simulink model "Second_AGC"  (R2022a)
settings: Solver=FixedStepDiscrete  StartTime=0.0  StopTime=Time*20000  RelTol=1e-3
PreLoadFcn:
  | clc,clear,close all
  | 
  | F               = 1e1;
  | Fs              = 200e6;
  | Frame           = 1  ;
  | Amplitudes      = [0.1,1,0.5,1,0.25];
  | R               = 2;
  | a               = 0.01;
  | alpha           = 0.4;
  | NumFrames       = length(Amplitudes);
  | SamplesY        = [];
  | TimeAxis        = [];
  | NumSym          = 1e3;
  | NumBitsInSymbol = 4;
  | sps             = 4;
  | rolloff         = 0.3;
  | span            = 32;
  | 
  | SQRRC = rcosdesign(rolloff, span, sps);
  | delay = mean(grpdelay(SQRRC));
  | for i = 1:NumFrames
  |     x = randi([0 3],NumSym,1);
  |     QPSK   = qammod(x,NumBitsInSymbol);
  |     Signal = Amplitudes(i) * upfirdn(QPSK, SQRRC, sps);
  |      Signal(1:delay-1)     = [];
  |      Signal(end-delay+3:end) = [];
  |     SamplesY = [SamplesY; Signal];
  | end
  | SamplesY = SamplesY.';
  | FixedRe = fi(real(SamplesY),1,16,14);
  | FixedIm = fi(imag(SamplesY),1,16,14);
  | FixedR  = fi(R,0,2,0);
  | Fixeda  = fi(a,1,13,12);
  | RealSimpleAGC = real(SamplesY);
  | ImagSimpleAGC = imag(SamplesY);
InitFcn:
  | Time = 40;
  | PowerDelay = Time*100;
libraries: sim_stud_lib_r2022a x25, dspsrcs4 x14, dspsigops x10, dspswit3 x5
(part 1 of 2)
settings Model: Creator=RolePups  LastModifiedBy=RolePups

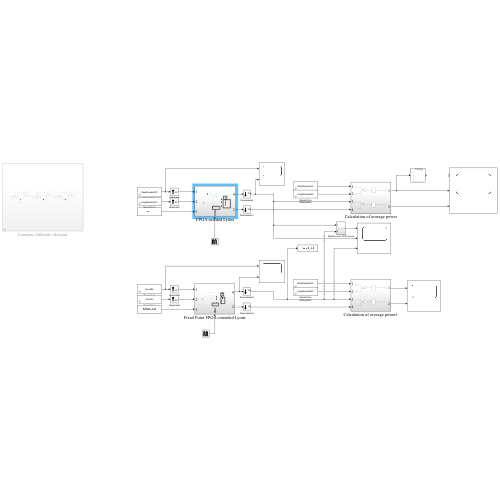
[thumbnail: Simulink's stored preview of the top-level diagram]
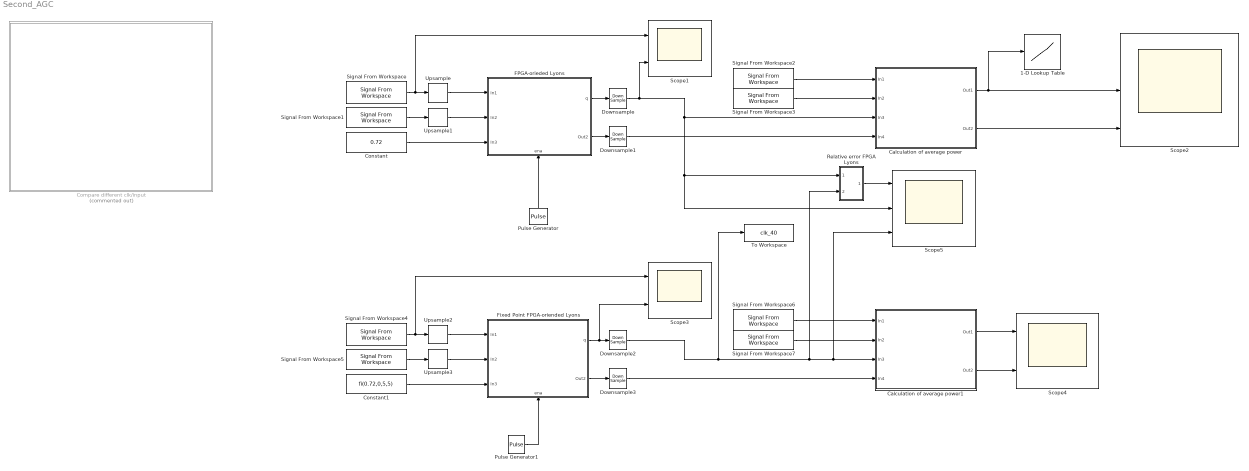
== system Second_AGC ==
  1-D Lookup Table : Lookup_n-D  NumberOfTableDimensions=1  BreakpointsForDimension1=[-5:5]  Table=10*log10([-5:5])  InternalRulePriority=Speed  RndMeth=Simplest
  Calculation of average power : Subsystem
  Calculation of average power1 : Subsystem
  Compare different clk/input : Subsystem  Commented=on
  Constant : Constant  Value=0.72
  Constant1 : Constant  Value=fi(0.72,0,5,5)
  Downsample{,1..3} (4 alike) : DownSample  N=Time  RateOptions=Allow multirate processing
  FPGA-orieded Lyons : Subsystem
      settings: PortSchema="{\"entries\":[{\"content\":{\"sides\":[{\"content\":{\"connectorIds\":[\"In1\",\"In2\",\"In3\"]},\"type\":\"ConnectorPlacement.EquallySpacedRectSide\",\"uuid\":\"2382ef4f-8b23-4fd9-9999-ae4ff3838c30\"},{\"content\":{\"connectorIds\":[\"Out1\",\"Out2\"],\"side\":\"RIGHT\"},\"type\":\"ConnectorPlacement.EquallySpacedRectSide\",\"uuid\":\"ff744322-ad90-46d9-948c-0637f52c7b9c\"},{\"content\":{\"connectorIds\":[],\"side\":\"TOP\"},\"type\":\"ConnectorPlacement.EquallySpacedRectSide\",\"uuid\":\"b0276f26-9e78-4e39-abf6-7a1348b88309\"},{\"content\":{\"connectorIds\":[\"In4\"],\"side\":\"BOTTOM\"},\"type\":\"ConnectorPlacement.EquallySpacedRectSide\",\"uuid\":\"b0dd70ff-8907-4b14-a46e-e3bbf4bdcae4\"}]},\"type\":\"ConnectorPlacement.EquallySpacedConnector\",\"uuid\":\"3f5cde89-4d4f-4bf7-b554-70cc79020603\"}],\"packageUris\":[\"http://schema.mathworks.com/mf0/Connector/R2020b\"],\"version\":\"1.0\"}"
  Fixed Point FPGA-oriended Lyons : Subsystem
      settings: PortSchema="{\"entries\":[{\"content\":{\"sides\":[{\"content\":{\"connectorIds\":[\"In1\",\"In2\",\"In3\"]},\"type\":\"ConnectorPlacement.EquallySpacedRectSide\",\"uuid\":\"2382ef4f-8b23-4fd9-9999-ae4ff3838c30\"},{\"content\":{\"connectorIds\":[\"Out1\",\"Out2\"],\"side\":\"RIGHT\"},\"type\":\"ConnectorPlacement.EquallySpacedRectSide\",\"uuid\":\"ff744322-ad90-46d9-948c-0637f52c7b9c\"},{\"content\":{\"connectorIds\":[],\"side\":\"TOP\"},\"type\":\"ConnectorPlacement.EquallySpacedRectSide\",\"uuid\":\"b0276f26-9e78-4e39-abf6-7a1348b88309\"},{\"content\":{\"connectorIds\":[\"In4\"],\"side\":\"BOTTOM\"},\"type\":\"ConnectorPlacement.EquallySpacedRectSide\",\"uuid\":\"b0dd70ff-8907-4b14-a46e-e3bbf4bdcae4\"}]},\"type\":\"ConnectorPlacement.EquallySpacedConnector\",\"uuid\":\"3f5cde89-4d4f-4bf7-b554-70cc79020603\"}],\"packageUris\":[\"http://schema.mathworks.com/mf0/Connector/R2020b\"],\"version\":\"1.0\"}"
  Pulse Generator : DiscretePulseGenerator  PulseType=Time based  Period=Time  PulseWidth=1/Time*100
  Pulse Generator1 : DiscretePulseGenerator  PulseType=Time based  Period=Time  PulseWidth=1/Time*100
  Relative error FPGA Lyons : Subsystem
  Scope1 : Scope  NumInputPorts=2
  Scope2 : Scope  NumInputPorts=3
  Scope3 : Scope  NumInputPorts=2
  Scope4 : Scope  NumInputPorts=2
  Scope5 : Scope  NumInputPorts=3
  Signal From Workspace : dspsrcs4/Signal From Workspace  X=RealSimpleAGC  Ts=Time  nsamps=1  OutputAfterFinalValue=Setting to zero  ignoreOrWarnInputAndFrameLengths=off  OutputFrames=off
  Signal From Workspace1 : dspsrcs4/Signal From Workspace  X=ImagSimpleAGC  Ts=Time  nsamps=1  OutputAfterFinalValue=Setting to zero  ignoreOrWarnInputAndFrameLengths=off  OutputFrames=off
  Signal From Workspace2 : dspsrcs4/Signal From Workspace  X=RealSimpleAGC  Ts=Time  nsamps=1  OutputAfterFinalValue=Setting to zero  ignoreOrWarnInputAndFrameLengths=off  OutputFrames=off
  Signal From Workspace3 : dspsrcs4/Signal From Workspace  X=ImagSimpleAGC  Ts=Time  nsamps=1  OutputAfterFinalValue=Setting to zero  ignoreOrWarnInputAndFrameLengths=off  OutputFrames=off
  Signal From Workspace4 : dspsrcs4/Signal From Workspace  X=FixedRe  Ts=Time  nsamps=1  OutputAfterFinalValue=Setting to zero  ignoreOrWarnInputAndFrameLengths=off  OutputFrames=off
  Signal From Workspace5 : dspsrcs4/Signal From Workspace  X=FixedIm  Ts=Time  nsamps=1  OutputAfterFinalValue=Setting to zero  ignoreOrWarnInputAndFrameLengths=off  OutputFrames=off
  Signal From Workspace6 : dspsrcs4/Signal From Workspace  X=RealSimpleAGC  Ts=Time  nsamps=1  OutputAfterFinalValue=Setting to zero  ignoreOrWarnInputAndFrameLengths=off  OutputFrames=off
  Signal From Workspace7 : dspsrcs4/Signal From Workspace  X=ImagSimpleAGC  Ts=Time  nsamps=1  OutputAfterFinalValue=Setting to zero  ignoreOrWarnInputAndFrameLengths=off  OutputFrames=off
  To Workspace : ToWorkspace  VariableName=clk_40  SampleTime=-1
  Upsample{,1..3} (4 alike) : dspsigops/Upsample  N=Time  phase=0  RateOptions=Allow multirate processing  ic=0  mode=Unused parameter value
  wires:
  Signal From Workspace/1 -> Scope1/1, Upsample/1
  Signal From Workspace1/1 -> Upsample1/1
  Upsample1/1 -> FPGA-orieded Lyons/2(In2)
  Constant/1 -> FPGA-orieded Lyons/3(In3)
  Pulse Generator/1 -> FPGA-orieded Lyons/4(ena)
  Upsample/1 -> FPGA-orieded Lyons/1(In1)
  FPGA-orieded Lyons/1(q) -> Downsample/1
  Downsample/1 -> Scope1/2, Scope5/2, Relative error FPGA Lyons/1(In1), Calculation of average power/3(In3)
  Signal From Workspace2/1 -> Calculation of average power/1(In1)
  Signal From Workspace3/1 -> Calculation of average power/2(In2)
  Calculation of average power/1(Out1) -> 1-D Lookup Table/1, Scope2/2
  FPGA-orieded Lyons/2(Out2) -> Downsample1/1
  Downsample1/1 -> Calculation of average power/4(In4)
  Calculation of average power/2(Out2) -> Scope2/3
  Signal From Workspace6/1 -> Calculation of average power1/1(In1)
  Signal From Workspace5/1 -> Upsample3/1
  Upsample3/1 -> Fixed Point FPGA-oriended Lyons/2(In2)
  Signal From Workspace4/1 -> Scope3/1, Upsample2/1
  Downsample3/1 -> Calculation of average power1/4(In4)
  Upsample2/1 -> Fixed Point FPGA-oriended Lyons/1(In1)
  Downsample2/1 -> To Workspace/1, Relative error FPGA Lyons/2(In3), Scope5/3, Calculation of average power1/3(In3)
  Calculation of average power1/2(Out2) -> Scope4/2
  Calculation of average power1/1(Out1) -> Scope4/1
  Fixed Point FPGA-oriended Lyons/1(q) -> Scope3/2, Downsample2/1
  Fixed Point FPGA-oriended Lyons/2(Out2) -> Downsample3/1
  Pulse Generator1/1 -> Fixed Point FPGA-oriended Lyons/4(ena)
  Constant1/1 -> Fixed Point FPGA-oriended Lyons/3(In3)
  Signal From Workspace7/1 -> Calculation of average power1/2(In2)
  Relative error FPGA Lyons/1(Out1) -> Scope5/1

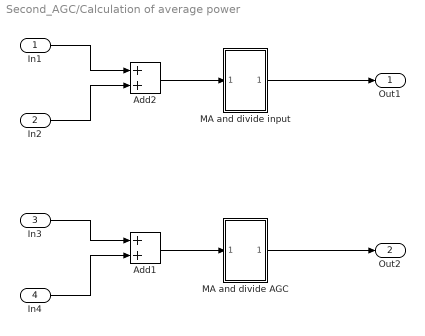
== system Second_AGC/Calculation of average power ==
  In1 : Inport
  In2 : Inport  Port=2
  In3 : Inport  Port=3
  In4 : Inport  Port=4
  Add1 : Sum
  Add2 : Sum
  MA and divide AGC : Subsystem
  "MA and divide input " : Subsystem
  Out1 : Outport
  Out2 : Outport  Port=2
  wires:
  In2/1 -> Add2/2
  In1/1 -> Add2/1
  In3/1 -> Add1/1
  In4/1 -> Add1/2
  Add1/1 -> MA and divide AGC/1(In2)
  MA and divide AGC/1(Out2) -> Out2/1
  "MA and divide input "/1(Out2) -> Out1/1
  Add2/1 -> "MA and divide input "/1(In2)

== system Second_AGC/Calculation of average power1 ==
  In1 : Inport
  In2 : Inport  Port=2
  In3 : Inport  Port=3
  In4 : Inport  Port=4
  Add1 : Sum
  Add2 : Sum
  MA and divide AGC : Subsystem
  "MA and divide input " : Subsystem
  Out1 : Outport
  Out2 : Outport  Port=2
  wires:
  In2/1 -> Add2/2
  In1/1 -> Add2/1
  In3/1 -> Add1/1
  In4/1 -> Add1/2
  Add1/1 -> MA and divide AGC/1(In2)
  MA and divide AGC/1(Out2) -> Out2/1
  "MA and divide input "/1(Out2) -> Out1/1
  Add2/1 -> "MA and divide input "/1(In2)

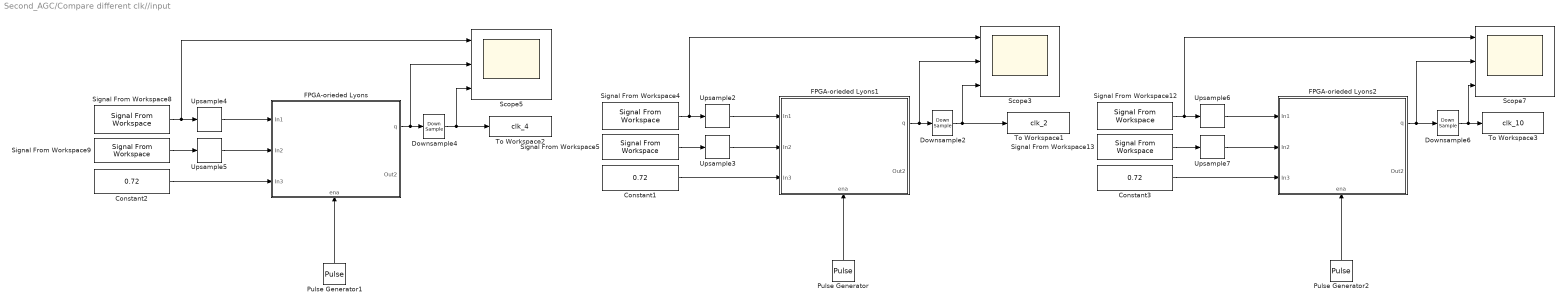
== system Second_AGC/Compare different clk//input ==
  Constant1 : Constant  Value=0.72
  Constant2 : Constant  Value=0.72
  Constant3 : Constant  Value=0.72
  Downsample2 : DownSample  RateOptions=Allow multirate processing
  Downsample4 : DownSample  N=4  RateOptions=Allow multirate processing
  Downsample6 : DownSample  N=10  RateOptions=Allow multirate processing
  FPGA-orieded Lyons : Subsystem
      settings: PortSchema="{\"entries\":[{\"content\":{\"sides\":[{\"content\":{\"connectorIds\":[\"In1\",\"In2\",\"In3\"]},\"type\":\"ConnectorPlacement.EquallySpacedRectSide\",\"uuid\":\"2382ef4f-8b23-4fd9-9999-ae4ff3838c30\"},{\"content\":{\"connectorIds\":[\"Out1\",\"Out2\"],\"side\":\"RIGHT\"},\"type\":\"ConnectorPlacement.EquallySpacedRectSide\",\"uuid\":\"ff744322-ad90-46d9-948c-0637f52c7b9c\"},{\"content\":{\"connectorIds\":[],\"side\":\"TOP\"},\"type\":\"ConnectorPlacement.EquallySpacedRectSide\",\"uuid\":\"b0276f26-9e78-4e39-abf6-7a1348b88309\"},{\"content\":{\"connectorIds\":[\"In4\"],\"side\":\"BOTTOM\"},\"type\":\"ConnectorPlacement.EquallySpacedRectSide\",\"uuid\":\"b0dd70ff-8907-4b14-a46e-e3bbf4bdcae4\"}]},\"type\":\"ConnectorPlacement.EquallySpacedConnector\",\"uuid\":\"3f5cde89-4d4f-4bf7-b554-70cc79020603\"}],\"packageUris\":[\"http://schema.mathworks.com/mf0/Connector/R2020b\"],\"version\":\"1.0\"}"
  FPGA-orieded Lyons1 : Subsystem
      settings: PortSchema="{\"entries\":[{\"content\":{\"sides\":[{\"content\":{\"connectorIds\":[\"In1\",\"In2\",\"In3\"]},\"type\":\"ConnectorPlacement.EquallySpacedRectSide\",\"uuid\":\"2382ef4f-8b23-4fd9-9999-ae4ff3838c30\"},{\"content\":{\"connectorIds\":[\"Out1\",\"Out2\"],\"side\":\"RIGHT\"},\"type\":\"ConnectorPlacement.EquallySpacedRectSide\",\"uuid\":\"ff744322-ad90-46d9-948c-0637f52c7b9c\"},{\"content\":{\"connectorIds\":[],\"side\":\"TOP\"},\"type\":\"ConnectorPlacement.EquallySpacedRectSide\",\"uuid\":\"b0276f26-9e78-4e39-abf6-7a1348b88309\"},{\"content\":{\"connectorIds\":[\"In4\"],\"side\":\"BOTTOM\"},\"type\":\"ConnectorPlacement.EquallySpacedRectSide\",\"uuid\":\"b0dd70ff-8907-4b14-a46e-e3bbf4bdcae4\"}]},\"type\":\"ConnectorPlacement.EquallySpacedConnector\",\"uuid\":\"3f5cde89-4d4f-4bf7-b554-70cc79020603\"}],\"packageUris\":[\"http://schema.mathworks.com/mf0/Connector/R2020b\"],\"version\":\"1.0\"}"
  FPGA-orieded Lyons2 : Subsystem
      settings: PortSchema="{\"entries\":[{\"content\":{\"sides\":[{\"content\":{\"connectorIds\":[\"In1\",\"In2\",\"In3\"]},\"type\":\"ConnectorPlacement.EquallySpacedRectSide\",\"uuid\":\"2382ef4f-8b23-4fd9-9999-ae4ff3838c30\"},{\"content\":{\"connectorIds\":[\"Out1\",\"Out2\"],\"side\":\"RIGHT\"},\"type\":\"ConnectorPlacement.EquallySpacedRectSide\",\"uuid\":\"ff744322-ad90-46d9-948c-0637f52c7b9c\"},{\"content\":{\"connectorIds\":[],\"side\":\"TOP\"},\"type\":\"ConnectorPlacement.EquallySpacedRectSide\",\"uuid\":\"b0276f26-9e78-4e39-abf6-7a1348b88309\"},{\"content\":{\"connectorIds\":[\"In4\"],\"side\":\"BOTTOM\"},\"type\":\"ConnectorPlacement.EquallySpacedRectSide\",\"uuid\":\"b0dd70ff-8907-4b14-a46e-e3bbf4bdcae4\"}]},\"type\":\"ConnectorPlacement.EquallySpacedConnector\",\"uuid\":\"3f5cde89-4d4f-4bf7-b554-70cc79020603\"}],\"packageUris\":[\"http://schema.mathworks.com/mf0/Connector/R2020b\"],\"version\":\"1.0\"}"
  Pulse Generator : DiscretePulseGenerator  PulseType=Time based  PulseWidth=50
  Pulse Generator1 : DiscretePulseGenerator  PulseType=Time based  Period=4  PulseWidth=25
  Pulse Generator2 : DiscretePulseGenerator  PulseType=Time based  Period=10  PulseWidth=10
  Scope3 : Scope  NumInputPorts=3
  Scope5 : Scope  NumInputPorts=3
  Scope7 : Scope  NumInputPorts=3
  Signal From Workspace12 : dspsrcs4/Signal From Workspace  X=RealSimpleAGC  Ts=10  nsamps=1  OutputAfterFinalValue=Setting to zero  ignoreOrWarnInputAndFrameLengths=off  OutputFrames=off
  Signal From Workspace13 : dspsrcs4/Signal From Workspace  X=ImagSimpleAGC  Ts=10  nsamps=1  OutputAfterFinalValue=Setting to zero  ignoreOrWarnInputAndFrameLengths=off  OutputFrames=off
  Signal From Workspace4 : dspsrcs4/Signal From Workspace  X=RealSimpleAGC  Ts=2  nsamps=1  OutputAfterFinalValue=Setting to zero  ignoreOrWarnInputAndFrameLengths=off  OutputFrames=off
  Signal From Workspace5 : dspsrcs4/Signal From Workspace  X=ImagSimpleAGC  Ts=2  nsamps=1  OutputAfterFinalValue=Setting to zero  ignoreOrWarnInputAndFrameLengths=off  OutputFrames=off
  Signal From Workspace8 : dspsrcs4/Signal From Workspace  X=RealSimpleAGC  Ts=4  nsamps=1  OutputAfterFinalValue=Setting to zero  ignoreOrWarnInputAndFrameLengths=off  OutputFrames=off
  Signal From Workspace9 : dspsrcs4/Signal From Workspace  X=ImagSimpleAGC  Ts=4  nsamps=1  OutputAfterFinalValue=Setting to zero  ignoreOrWarnInputAndFrameLengths=off  OutputFrames=off
  To Workspace1 : ToWorkspace  VariableName=clk_2  SampleTime=-1
  To Workspace2 : ToWorkspace  VariableName=clk_4  SampleTime=-1
  To Workspace3 : ToWorkspace  VariableName=clk_10  SampleTime=-1
  Upsample2 : dspsigops/Upsample  N=2  phase=0  RateOptions=Allow multirate processing  ic=0  mode=Unused parameter value
  Upsample3 : dspsigops/Upsample  N=2  phase=0  RateOptions=Allow multirate processing  ic=0  mode=Unused parameter value
  Upsample4 : dspsigops/Upsample  N=4  phase=0  RateOptions=Allow multirate processing  ic=0  mode=Unused parameter value
  Upsample5 : dspsigops/Upsample  N=4  phase=0  RateOptions=Allow multirate processing  ic=0  mode=Unused parameter value
  Upsample6 : dspsigops/Upsample  N=10  phase=0  RateOptions=Allow multirate processing  ic=0  mode=Unused parameter value
  Upsample7 : dspsigops/Upsample  N=10  phase=0  RateOptions=Allow multirate processing  ic=0  mode=Unused parameter value
  wires:
  Downsample4/1 -> Scope5/3, To Workspace2/1
  FPGA-orieded Lyons1/1(q) -> Scope3/2, Downsample2/1
  Upsample4/1 -> FPGA-orieded Lyons/1(In1)
  Signal From Workspace9/1 -> Upsample5/1
  Signal From Workspace8/1 -> Scope5/1, Upsample4/1
  Signal From Workspace4/1 -> Scope3/1, Upsample2/1
  Downsample2/1 -> Scope3/3, To Workspace1/1
  Signal From Workspace5/1 -> Upsample3/1
  Upsample6/1 -> FPGA-orieded Lyons2/1(In1)
  Upsample5/1 -> FPGA-orieded Lyons/2(In2)
  FPGA-orieded Lyons/1(q) -> Scope5/2, Downsample4/1
  Signal From Workspace12/1 -> Scope7/1, Upsample6/1
  Constant3/1 -> FPGA-orieded Lyons2/3(In3)
  Signal From Workspace13/1 -> Upsample7/1
  Upsample7/1 -> FPGA-orieded Lyons2/2(In2)
  Constant2/1 -> FPGA-orieded Lyons/3(In3)
  Downsample6/1 -> Scope7/3, To Workspace3/1
  Upsample2/1 -> FPGA-orieded Lyons1/1(In1)
  Upsample3/1 -> FPGA-orieded Lyons1/2(In2)
  Constant1/1 -> FPGA-orieded Lyons1/3(In3)
  FPGA-orieded Lyons2/1(q) -> Scope7/2, Downsample6/1
  Pulse Generator1/1 -> FPGA-orieded Lyons/4(ena)
  Pulse Generator/1 -> FPGA-orieded Lyons1/4(ena)
  Pulse Generator2/1 -> FPGA-orieded Lyons2/4(ena)

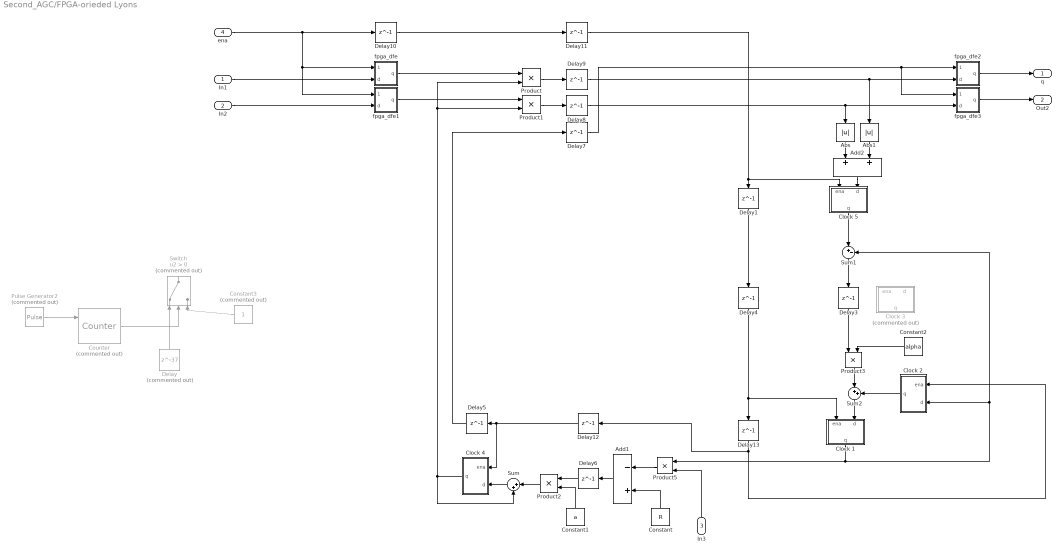
== system Second_AGC/FPGA-orieded Lyons ==
  In1 : Inport
  In2 : Inport  Port=2
  In3 : Inport  Port=3
  ena : Inport  Port=4
  Abs : Abs  SaturateOnIntegerOverflow=off
  Abs1 : Abs  SaturateOnIntegerOverflow=off
  Add1 : Sum  Inputs=-+  AccumDataTypeStr=double
  Add2 : Sum  AccumDataTypeStr=double
  Clock 1 : Subsystem
  Clock 2 : Subsystem
  Clock 3 : Subsystem  Commented=on
  Clock 4 : Subsystem
  Clock 5 : Subsystem
  Constant : Constant  Value=R  SampleTime=-1
  Constant1 : Constant  Value=a  SampleTime=-1
  Constant2 : Constant  Value=alpha  SampleTime=-1
  Constant3 : Constant  Commented=on  SampleTime=-1
  Counter : dspswit3/Counter  Commented=on  Direction=Up  CountEvent=Rising edge  CounterSize=User defined  MaxCount=1  InitialCount=0  Output=Count  HitValue=32  ResetInput=on  SamplesPerFrame=1  Ts=1  CntDtype=double  HitDtype=Logical
  Delay : Delay  Commented=on  DelayLength=37  InitialCondition=0
  Delay{1,3..13} (12 alike) : Delay  DelayLength=1  InitialCondition=0
  Product{,1..3,5} (5 alike) : Product  OutDataTypeStr=double
  Pulse Generator2 : DiscretePulseGenerator  Commented=on  PulseType=Time based  Period=Time*20000  PulseWidth=50  PhaseDelay=41
  Sum : Sum  Inputs=|++  AccumDataTypeStr=double
  Sum1 : Sum  Inputs=|+-  AccumDataTypeStr=double
  Sum2 : Sum  Inputs=|++  AccumDataTypeStr=double
  Switch : Switch  Commented=on  Criteria=u2 > Threshold  SaturateOnIntegerOverflow=off  InputSameDT=off
  fpga_dfe : Subsystem  AncestorBlock=sim_stud_lib_r2022a/fpga_dfe
      mask Display:
      | disp('D');
      | port_label('input',1,'e');
      | port_label('input',2,'d');
      | port_label('output',1,'q');
  fpga_dfe1 : Subsystem  AncestorBlock=sim_stud_lib_r2022a/fpga_dfe
      mask Display:
      | disp('D');
      | port_label('input',1,'e');
      | port_label('input',2,'d');
      | port_label('output',1,'q');
  fpga_dfe2 : Subsystem  AncestorBlock=sim_stud_lib_r2022a/fpga_dfe
      mask Display:
      | disp('D');
      | port_label('input',1,'e');
      | port_label('input',2,'d');
      | port_label('output',1,'q');
  fpga_dfe3 : Subsystem  AncestorBlock=sim_stud_lib_r2022a/fpga_dfe
      mask Display:
      | disp('D');
      | port_label('input',1,'e');
      | port_label('input',2,'d');
      | port_label('output',1,'q');
  q : Outport
  Out2 : Outport  Port=2
  wires:
  Clock 4/1(q) -> Sum/2, Product1/2, Product/2
  Product/1 -> Delay9/1
  Product1/1 -> Delay8/1
  Constant/1 -> Add1/2
  Sum/1 -> Clock 4/2(d)
  Product2/1 -> Sum/1
  Constant1/1 -> Product2/2
  Abs1/1 -> Add2/2
  Abs/1 -> Add2/1
  In3/1 -> Product5/2
  Product5/1 -> Add1/1
  Constant2/1 -> Product3/2
  Product3/1 -> Sum2/1
  Clock 2/1(q) -> Sum2/2
  fpga_dfe/1(q) -> Product/1
  fpga_dfe1/1(q) -> Product1/1
  Add1/1 -> Delay6/1
  Constant3/1 -> Switch/3
  Counter/1 -> Switch/2
  Pulse Generator2/1 -> Counter/1
  Sum2/1 -> Clock 1/2(d)
  Clock 1/1(q) -> Product5/1, Sum1/2, Clock 2/2(d)
  Delay/1 -> Switch/1
  fpga_dfe2/1(q) -> q/1
  fpga_dfe3/1(q) -> Out2/1
  Add2/1 -> Clock 5/2(d)
  Clock 5/1(q) -> Sum1/1
  In1/1 -> fpga_dfe/2(d)
  In2/1 -> fpga_dfe1/2(d)
  Delay8/1 -> fpga_dfe3/2(d), Abs/1
  Delay9/1 -> Abs1/1, fpga_dfe2/2(d)
  Sum1/1 -> Delay3/1
  Delay3/1 -> Product3/1
  Delay4/1 -> Delay13/1, Clock 1/1(ena)
  Delay13/1 -> Clock 2/1(ena), Delay12/1
  Delay6/1 -> Product2/1
  Delay5/1 -> Delay7/1
  Delay7/1 -> fpga_dfe3/1(ena), fpga_dfe2/1(ena)
  ena/1 -> Delay10/1, fpga_dfe1/1(ena), fpga_dfe/1(ena)
  Delay10/1 -> Delay11/1
  Delay11/1 -> Clock 5/1(ena), Delay1/1
  Delay1/1 -> Delay4/1
  Delay12/1 -> Clock 4/1(ena), Delay5/1

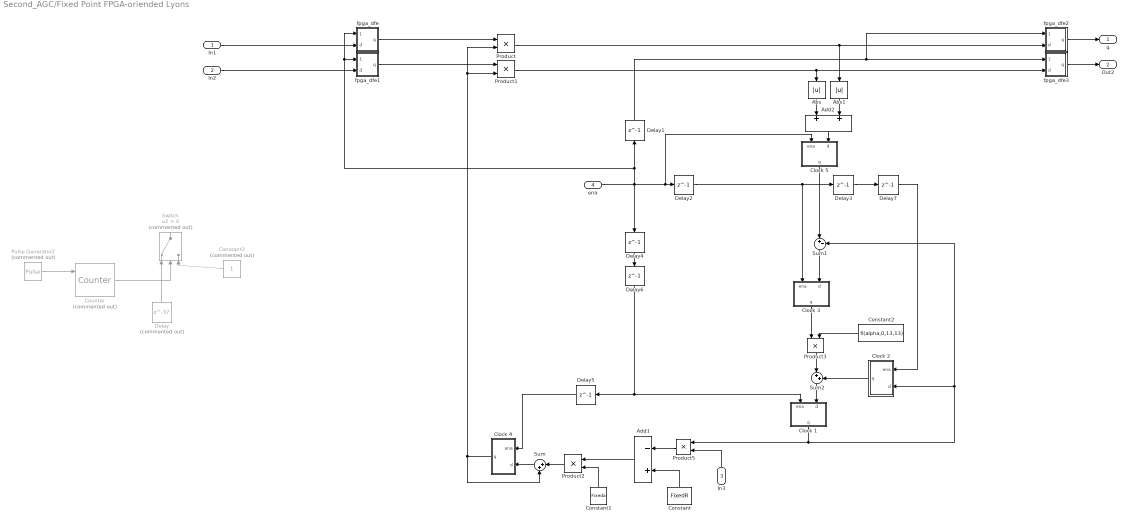
== system Second_AGC/Fixed Point FPGA-oriended Lyons ==
  In1 : Inport
  In2 : Inport  Port=2
  In3 : Inport  Port=3
  ena : Inport  Port=4
  Abs : Abs  OutDataTypeStr=fixdt(0,26,20)  SaturateOnIntegerOverflow=off
  Abs1 : Abs  OutDataTypeStr=fixdt(0,26,20)  SaturateOnIntegerOverflow=off
  Add1 : Sum  Inputs=-+  AccumDataTypeStr=fixdt(1,27,18)  OutDataTypeStr=fixdt(1,27,18)
  Add2 : Sum  AccumDataTypeStr=fixdt(0,27,18)  OutDataTypeStr=fixdt(0,27,18)
  Clock 1 : Subsystem
  Clock 2 : Subsystem
  Clock 3 : Subsystem
  Clock 4 : Subsystem
  Clock 5 : Subsystem
  Constant : Constant  Value=FixedR  SampleTime=-1
  Constant1 : Constant  Value=Fixeda  SampleTime=-1
  Constant2 : Constant  Value=fi(alpha,0,13,13)  SampleTime=-1
  Constant3 : Constant  Commented=on  SampleTime=-1
  Counter : dspswit3/Counter  Commented=on  Direction=Up  CountEvent=Rising edge  CounterSize=User defined  MaxCount=1  InitialCount=0  Output=Count  HitValue=32  ResetInput=on  SamplesPerFrame=1  Ts=1  CntDtype=double  HitDtype=Logical
  Delay : Delay  Commented=on  DelayLength=37  InitialCondition=0
  Delay{1..7} (7 alike) : Delay  DelayLength=1  InitialCondition=0
  Product : Product  OutDataTypeStr=fixdt(1,26,18)
  Product1 : Product  OutDataTypeStr=fixdt(1,26,18)
  Product2 : Product  OutDataTypeStr=fixdt(1,41,33)
  Product3 : Product  OutDataTypeStr=fixdt(1,48,32)
  Product5 : Product  OutDataTypeStr=fixdt(1,27,18)
  Pulse Generator2 : DiscretePulseGenerator  Commented=on  PulseType=Time based  Period=Time*20000  PulseWidth=50  PhaseDelay=41
  Sum : Sum  Inputs=|++  AccumDataTypeStr=fixdt(1,48,32)  OutDataTypeStr=fixdt(1,48,32)
  Sum1 : Sum  Inputs=|+-  AccumDataTypeStr=fixdt(1,27,18)  OutDataTypeStr=fixdt(1,27,18)
  Sum2 : Sum  Inputs=|++  AccumDataTypeStr=fixdt(1,48,32)  OutDataTypeStr=fixdt(1,48,32)
  Switch : Switch  Commented=on  Criteria=u2 > Threshold  SaturateOnIntegerOverflow=off  InputSameDT=off
  fpga_dfe : Subsystem  AncestorBlock=sim_stud_lib_r2022a/fpga_dfe
      mask Display:
      | disp('D');
      | port_label('input',1,'e');
      | port_label('input',2,'d');
      | port_label('output',1,'q');
  fpga_dfe1 : Subsystem  AncestorBlock=sim_stud_lib_r2022a/fpga_dfe
      mask Display:
      | disp('D');
      | port_label('input',1,'e');
      | port_label('input',2,'d');
      | port_label('output',1,'q');
  fpga_dfe2 : Subsystem  AncestorBlock=sim_stud_lib_r2022a/fpga_dfe
      mask Display:
      | disp('D');
      | port_label('input',1,'e');
      | port_label('input',2,'d');
      | port_label('output',1,'q');
  fpga_dfe3 : Subsystem  AncestorBlock=sim_stud_lib_r2022a/fpga_dfe
      mask Display:
      | disp('D');
      | port_label('input',1,'e');
      | port_label('input',2,'d');
      | port_label('output',1,'q');
  q : Outport
  Out2 : Outport  Port=2
  wires:
  Clock 4/1(q) -> Sum/2, Product/2, Product1/2
  Product/1 -> fpga_dfe2/2(d), Abs1/1
  Product1/1 -> fpga_dfe3/2(d), Abs/1
  Constant/1 -> Add1/2
  Sum/1 -> Clock 4/2(d)
  Product2/1 -> Sum/1
  Constant1/1 -> Product2/2
  Abs1/1 -> Add2/2
  Abs/1 -> Add2/1
  In3/1 -> Product5/2
  Sum1/1 -> Clock 3/2(d)
  Product5/1 -> Add1/1
  Constant2/1 -> Product3/2
  Product3/1 -> Sum2/1
  Clock 2/1(q) -> Sum2/2
  fpga_dfe/1(q) -> Product/1
  fpga_dfe1/1(q) -> Product1/1
  Add1/1 -> Product2/1
  Constant3/1 -> Switch/3
  Counter/1 -> Switch/2
  Pulse Generator2/1 -> Counter/1
  Sum2/1 -> Clock 1/2(d)
  Clock 1/1(q) -> Product5/1, Sum1/2, Clock 2/2(d)
  Clock 3/1(q) -> Product3/1
  Delay/1 -> Switch/1
  fpga_dfe2/1(q) -> q/1
  fpga_dfe3/1(q) -> Out2/1
  ena/1 -> Delay4/1, Delay1/1, fpga_dfe1/1(ena), fpga_dfe/1(ena), Clock 5/1(ena), Delay2/1
  Delay2/1 -> Delay3/1, Clock 3/1(ena)
  Delay3/1 -> Delay7/1
  Delay4/1 -> Delay6/1
  Delay5/1 -> Clock 4/1(ena)
  Delay7/1 -> Clock 2/1(ena)
  Add2/1 -> Clock 5/2(d)
  Clock 5/1(q) -> Sum1/1
  In1/1 -> fpga_dfe/2(d)
  In2/1 -> fpga_dfe1/2(d)
  Delay6/1 -> Clock 1/1(ena), Delay5/1
  Delay1/1 -> fpga_dfe3/1(ena), fpga_dfe2/1(ena)

== system Second_AGC/Relative error FPGA Lyons ==
  In1 : Inport
  In3 : Inport  Port=2
  Add1 : Sum  Inputs=-+  AccumDataTypeStr=double
  Divide : Product  Inputs=*/
  Out1 : Outport
  wires:
  Add1/1 -> Divide/1
  In3/1 -> Divide/2, Add1/2
  Divide/1 -> Out1/1
  In1/1 -> Add1/1

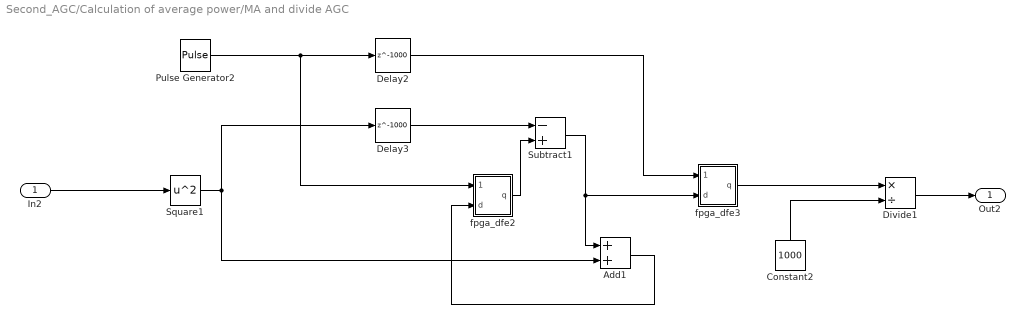
== system Second_AGC/Calculation of average power/MA and divide AGC ==
  In2 : Inport
  Add1 : Sum
  Constant2 : Constant  Value=1000
  Delay2 : Delay  DelayLength=1000
  Delay3 : Delay  DelayLength=1000
  Divide1 : Product  Inputs=*/
  Pulse Generator2 : DiscretePulseGenerator  PulseType=Time based  Period=Time  PulseWidth=1/Time*100
  Square1 : Math  Operator=square
  Subtract1 : Sum  Inputs=-+
  fpga_dfe2 : Subsystem  AncestorBlock=sim_stud_lib_r2022a/fpga_dfe
      mask Display:
      | disp('D');
      | port_label('input',1,'e');
      | port_label('input',2,'d');
      | port_label('output',1,'q');
  fpga_dfe3 : Subsystem  AncestorBlock=sim_stud_lib_r2022a/fpga_dfe
      mask Display:
      | disp('D');
      | port_label('input',1,'e');
      | port_label('input',2,'d');
      | port_label('output',1,'q');
  Out2 : Outport
  wires:
  Divide1/1 -> Out2/1
  fpga_dfe3/1(q) -> Divide1/1
  Delay3/1 -> Subtract1/1
  Add1/1 -> fpga_dfe2/2(d)
  Constant2/1 -> Divide1/2
  Subtract1/1 -> Add1/1, fpga_dfe3/2(d)
  Square1/1 -> Add1/2, Delay3/1
  fpga_dfe2/1(q) -> Subtract1/2
  Delay2/1 -> fpga_dfe3/1(ena)
  In2/1 -> Square1/1
  Pulse Generator2/1 -> fpga_dfe2/1(ena), Delay2/1

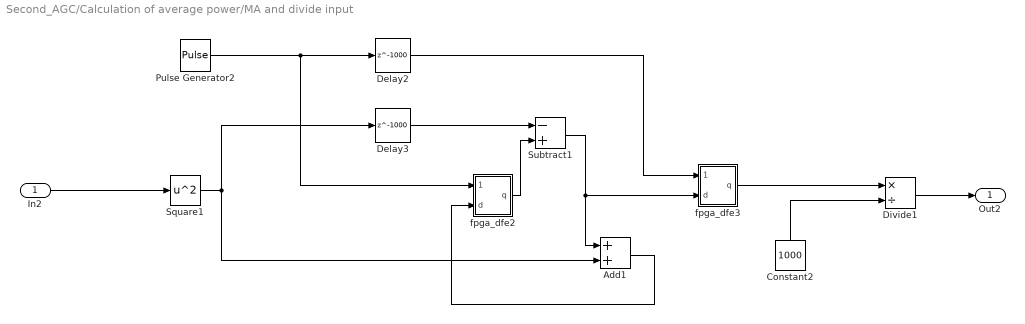
== system Second_AGC/Calculation of average power/MA and divide input  ==
  In2 : Inport
  Add1 : Sum
  Constant2 : Constant  Value=1000
  Delay2 : Delay  DelayLength=1000
  Delay3 : Delay  DelayLength=1000
  Divide1 : Product  Inputs=*/
  Pulse Generator2 : DiscretePulseGenerator  PulseType=Time based  Period=Time  PulseWidth=1/Time*100
  Square1 : Math  Operator=square
  Subtract1 : Sum  Inputs=-+
  fpga_dfe2 : Subsystem  AncestorBlock=sim_stud_lib_r2022a/fpga_dfe
      mask Display:
      | disp('D');
      | port_label('input',1,'e');
      | port_label('input',2,'d');
      | port_label('output',1,'q');
  fpga_dfe3 : Subsystem  AncestorBlock=sim_stud_lib_r2022a/fpga_dfe
      mask Display:
      | disp('D');
      | port_label('input',1,'e');
      | port_label('input',2,'d');
      | port_label('output',1,'q');
  Out2 : Outport
  wires:
  Divide1/1 -> Out2/1
  fpga_dfe3/1(q) -> Divide1/1
  Delay3/1 -> Subtract1/1
  Add1/1 -> fpga_dfe2/2(d)
  Constant2/1 -> Divide1/2
  Subtract1/1 -> Add1/1, fpga_dfe3/2(d)
  Square1/1 -> Add1/2, Delay3/1
  fpga_dfe2/1(q) -> Subtract1/2
  Delay2/1 -> fpga_dfe3/1(ena)
  In2/1 -> Square1/1
  Pulse Generator2/1 -> fpga_dfe2/1(ena), Delay2/1

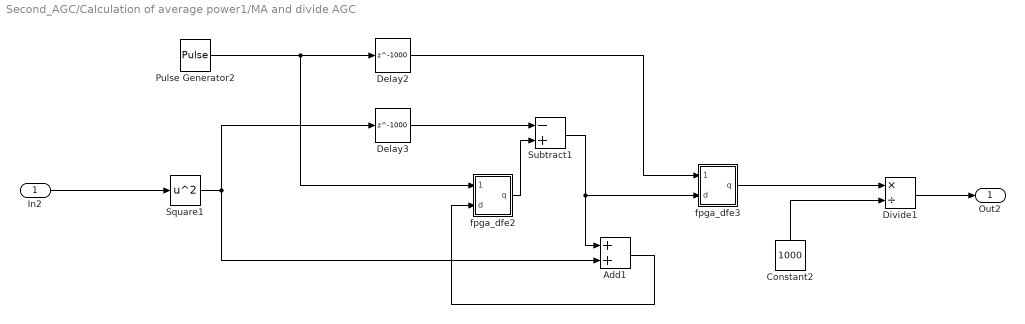
== system Second_AGC/Calculation of average power1/MA and divide AGC ==
  In2 : Inport
  Add1 : Sum
  Constant2 : Constant  Value=1000
  Delay2 : Delay  DelayLength=1000
  Delay3 : Delay  DelayLength=1000
  Divide1 : Product  Inputs=*/
  Pulse Generator2 : DiscretePulseGenerator  PulseType=Time based  Period=Time  PulseWidth=1/Time*100
  Square1 : Math  Operator=square
  Subtract1 : Sum  Inputs=-+
  fpga_dfe2 : Subsystem  AncestorBlock=sim_stud_lib_r2022a/fpga_dfe
      mask Display:
      | disp('D');
      | port_label('input',1,'e');
      | port_label('input',2,'d');
      | port_label('output',1,'q');
  fpga_dfe3 : Subsystem  AncestorBlock=sim_stud_lib_r2022a/fpga_dfe
      mask Display:
      | disp('D');
      | port_label('input',1,'e');
      | port_label('input',2,'d');
      | port_label('output',1,'q');
  Out2 : Outport
  wires:
  Divide1/1 -> Out2/1
  fpga_dfe3/1(q) -> Divide1/1
  Delay3/1 -> Subtract1/1
  Add1/1 -> fpga_dfe2/2(d)
  Constant2/1 -> Divide1/2
  Subtract1/1 -> Add1/1, fpga_dfe3/2(d)
  Square1/1 -> Add1/2, Delay3/1
  fpga_dfe2/1(q) -> Subtract1/2
  Delay2/1 -> fpga_dfe3/1(ena)
  In2/1 -> Square1/1
  Pulse Generator2/1 -> fpga_dfe2/1(ena), Delay2/1

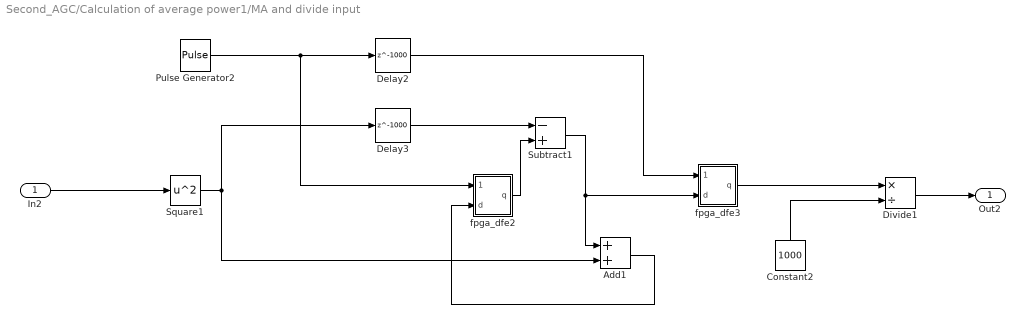
== system Second_AGC/Calculation of average power1/MA and divide input  ==
  In2 : Inport
  Add1 : Sum
  Constant2 : Constant  Value=1000
  Delay2 : Delay  DelayLength=1000
  Delay3 : Delay  DelayLength=1000
  Divide1 : Product  Inputs=*/
  Pulse Generator2 : DiscretePulseGenerator  PulseType=Time based  Period=Time  PulseWidth=1/Time*100
  Square1 : Math  Operator=square
  Subtract1 : Sum  Inputs=-+
  fpga_dfe2 : Subsystem  AncestorBlock=sim_stud_lib_r2022a/fpga_dfe
      mask Display:
      | disp('D');
      | port_label('input',1,'e');
      | port_label('input',2,'d');
      | port_label('output',1,'q');
  fpga_dfe3 : Subsystem  AncestorBlock=sim_stud_lib_r2022a/fpga_dfe
      mask Display:
      | disp('D');
      | port_label('input',1,'e');
      | port_label('input',2,'d');
      | port_label('output',1,'q');
  Out2 : Outport
  wires:
  Divide1/1 -> Out2/1
  fpga_dfe3/1(q) -> Divide1/1
  Delay3/1 -> Subtract1/1
  Add1/1 -> fpga_dfe2/2(d)
  Constant2/1 -> Divide1/2
  Subtract1/1 -> Add1/1, fpga_dfe3/2(d)
  Square1/1 -> Add1/2, Delay3/1
  fpga_dfe2/1(q) -> Subtract1/2
  Delay2/1 -> fpga_dfe3/1(ena)
  In2/1 -> Square1/1
  Pulse Generator2/1 -> fpga_dfe2/1(ena), Delay2/1

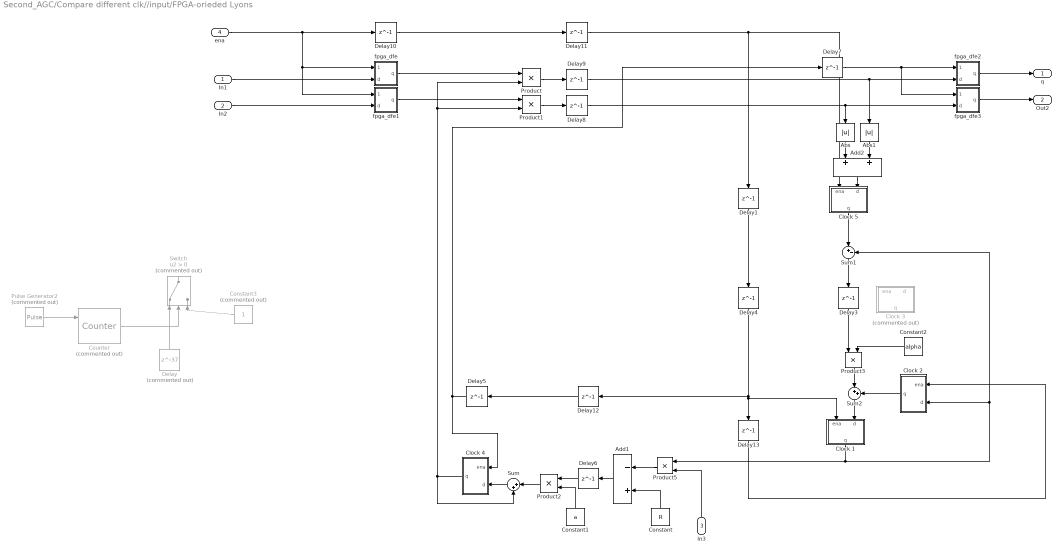
== system Second_AGC/Compare different clk//input/FPGA-orieded Lyons ==
  In1 : Inport
  In2 : Inport  Port=2
  In3 : Inport  Port=3
  ena : Inport  Port=4
  Abs : Abs  SaturateOnIntegerOverflow=off
  Abs1 : Abs  SaturateOnIntegerOverflow=off
  Add1 : Sum  Inputs=-+  AccumDataTypeStr=double
  Add2 : Sum  AccumDataTypeStr=double
  Clock 1 : Subsystem
  Clock 2 : Subsystem
  Clock 3 : Subsystem  Commented=on
  Clock 4 : Subsystem
  Clock 5 : Subsystem
  Constant : Constant  Value=R  SampleTime=-1
  Constant1 : Constant  Value=a  SampleTime=-1
  Constant2 : Constant  Value=alpha  SampleTime=-1
  Constant3 : Constant  Commented=on  SampleTime=-1
  Counter : dspswit3/Counter  Commented=on  Direction=Up  CountEvent=Rising edge  CounterSize=User defined  MaxCount=1  InitialCount=0  Output=Count  HitValue=32  ResetInput=on  SamplesPerFrame=1  Ts=1  CntDtype=double  HitDtype=Logical
  Delay : Delay  Commented=on  DelayLength=37  InitialCondition=0
  Delay{1,3..13} (12 alike) : Delay  DelayLength=1  InitialCondition=0
  Product{,1..3,5} (5 alike) : Product  OutDataTypeStr=double
  Pulse Generator2 : DiscretePulseGenerator  Commented=on  PulseType=Time based  Period=Time*20000  PulseWidth=50  PhaseDelay=41
  Sum : Sum  Inputs=|++  AccumDataTypeStr=double
  Sum1 : Sum  Inputs=|+-  AccumDataTypeStr=double
  Sum2 : Sum  Inputs=|++  AccumDataTypeStr=double
  Switch : Switch  Commented=on  Criteria=u2 > Threshold  SaturateOnIntegerOverflow=off  InputSameDT=off
  fpga_dfe : Subsystem  AncestorBlock=sim_stud_lib_r2022a/fpga_dfe
      mask Display:
      | disp('D');
      | port_label('input',1,'e');
      | port_label('input',2,'d');
      | port_label('output',1,'q');
  fpga_dfe1 : Subsystem  AncestorBlock=sim_stud_lib_r2022a/fpga_dfe
      mask Display:
      | disp('D');
      | port_label('input',1,'e');
      | port_label('input',2,'d');
      | port_label('output',1,'q');
  fpga_dfe2 : Subsystem  AncestorBlock=sim_stud_lib_r2022a/fpga_dfe
      mask Display:
      | disp('D');
      | port_label('input',1,'e');
      | port_label('input',2,'d');
      | port_label('output',1,'q');
  fpga_dfe3 : Subsystem  AncestorBlock=sim_stud_lib_r2022a/fpga_dfe
      mask Display:
      | disp('D');
      | port_label('input',1,'e');
      | port_label('input',2,'d');
      | port_label('output',1,'q');
  q : Outport
  Out2 : Outport  Port=2
  wires:
  Clock 4/1(q) -> Sum/2, Product1/2, Product/2
  Product/1 -> Delay9/1
  Product1/1 -> Delay8/1
  Constant/1 -> Add1/2
  Sum/1 -> Clock 4/2(d)
  Product2/1 -> Sum/1
  Constant1/1 -> Product2/2
  Abs1/1 -> Add2/2
  Abs/1 -> Add2/1
  In3/1 -> Product5/2
  Product5/1 -> Add1/1
  Constant2/1 -> Product3/2
  Product3/1 -> Sum2/1
  Clock 2/1(q) -> Sum2/2
  fpga_dfe/1(q) -> Product/1
  fpga_dfe1/1(q) -> Product1/1
  Add1/1 -> Delay6/1
  Constant3/1 -> Switch/3
  Counter/1 -> Switch/2
  Pulse Generator2/1 -> Counter/1
  Sum2/1 -> Clock 1/2(d)
  Clock 1/1(q) -> Product5/1, Sum1/2, Clock 2/2(d)
  Delay/1 -> Switch/1
  fpga_dfe2/1(q) -> q/1
  fpga_dfe3/1(q) -> Out2/1
  Add2/1 -> Clock 5/2(d)
  Clock 5/1(q) -> Sum1/1
  In1/1 -> fpga_dfe/2(d)
  In2/1 -> fpga_dfe1/2(d)
  Delay8/1 -> fpga_dfe3/2(d), Abs/1
  Delay9/1 -> Abs1/1, fpga_dfe2/2(d)
  Sum1/1 -> Delay3/1
  Delay3/1 -> Product3/1
  Delay4/1 -> Delay12/1, Delay13/1, Clock 1/1(ena)
  Delay13/1 -> Clock 2/1(ena)
  Delay6/1 -> Product2/1
  Delay5/1 -> Delay7/1, Clock 4/1(ena)
  Delay7/1 -> fpga_dfe3/1(ena), fpga_dfe2/1(ena)
  ena/1 -> Delay10/1, fpga_dfe1/1(ena), fpga_dfe/1(ena)
  Delay10/1 -> Delay11/1
  Delay11/1 -> Delay1/1, Clock 5/1(ena)
  Delay1/1 -> Delay4/1
  Delay12/1 -> Delay5/1

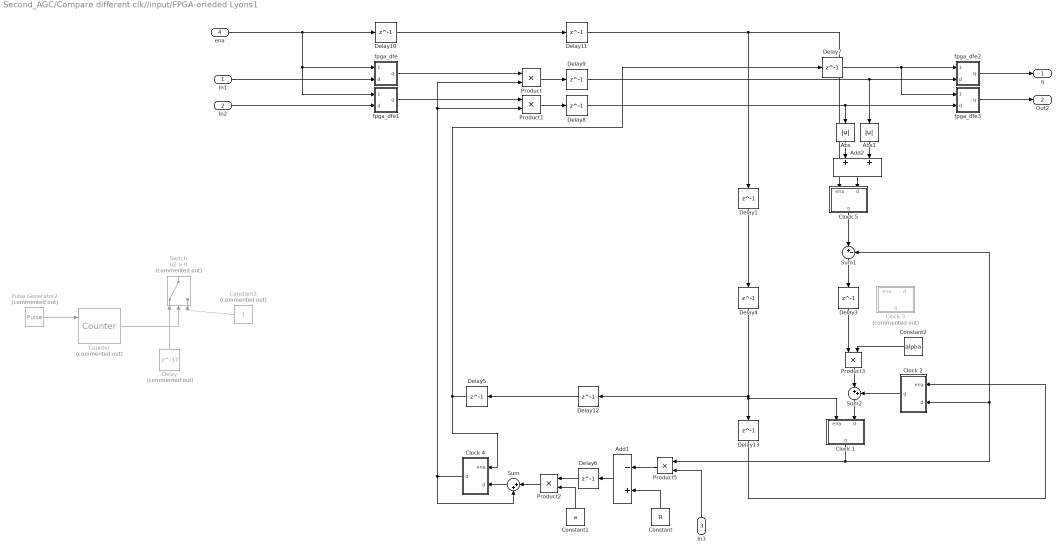
== system Second_AGC/Compare different clk//input/FPGA-orieded Lyons1 ==
  In1 : Inport
  In2 : Inport  Port=2
  In3 : Inport  Port=3
  ena : Inport  Port=4
  Abs : Abs  SaturateOnIntegerOverflow=off
  Abs1 : Abs  SaturateOnIntegerOverflow=off
  Add1 : Sum  Inputs=-+  AccumDataTypeStr=double
  Add2 : Sum  AccumDataTypeStr=double
  Clock 1 : Subsystem
  Clock 2 : Subsystem
  Clock 3 : Subsystem  Commented=on
  Clock 4 : Subsystem
  Clock 5 : Subsystem
  Constant : Constant  Value=R  SampleTime=-1
  Constant1 : Constant  Value=a  SampleTime=-1
  Constant2 : Constant  Value=alpha  SampleTime=-1
  Constant3 : Constant  Commented=on  SampleTime=-1
  Counter : dspswit3/Counter  Commented=on  Direction=Up  CountEvent=Rising edge  CounterSize=User defined  MaxCount=1  InitialCount=0  Output=Count  HitValue=32  ResetInput=on  SamplesPerFrame=1  Ts=1  CntDtype=double  HitDtype=Logical
  Delay : Delay  Commented=on  DelayLength=37  InitialCondition=0
  Delay{1,3..13} (12 alike) : Delay  DelayLength=1  InitialCondition=0
  Product{,1..3,5} (5 alike) : Product  OutDataTypeStr=double
  Pulse Generator2 : DiscretePulseGenerator  Commented=on  PulseType=Time based  Period=Time*20000  PulseWidth=50  PhaseDelay=41
  Sum : Sum  Inputs=|++  AccumDataTypeStr=double
  Sum1 : Sum  Inputs=|+-  AccumDataTypeStr=double
  Sum2 : Sum  Inputs=|++  AccumDataTypeStr=double
  Switch : Switch  Commented=on  Criteria=u2 > Threshold  SaturateOnIntegerOverflow=off  InputSameDT=off
  fpga_dfe : Subsystem  AncestorBlock=sim_stud_lib_r2022a/fpga_dfe
      mask Display:
      | disp('D');
      | port_label('input',1,'e');
      | port_label('input',2,'d');
      | port_label('output',1,'q');
  fpga_dfe1 : Subsystem  AncestorBlock=sim_stud_lib_r2022a/fpga_dfe
      mask Display:
      | disp('D');
      | port_label('input',1,'e');
      | port_label('input',2,'d');
      | port_label('output',1,'q');
  fpga_dfe2 : Subsystem  AncestorBlock=sim_stud_lib_r2022a/fpga_dfe
      mask Display:
      | disp('D');
      | port_label('input',1,'e');
      | port_label('input',2,'d');
      | port_label('output',1,'q');
  fpga_dfe3 : Subsystem  AncestorBlock=sim_stud_lib_r2022a/fpga_dfe
      mask Display:
      | disp('D');
      | port_label('input',1,'e');
      | port_label('input',2,'d');
      | port_label('output',1,'q');
  q : Outport
  Out2 : Outport  Port=2
  wires:
  Clock 4/1(q) -> Sum/2, Product1/2, Product/2
  Product/1 -> Delay9/1
  Product1/1 -> Delay8/1
  Constant/1 -> Add1/2
  Sum/1 -> Clock 4/2(d)
  Product2/1 -> Sum/1
  Constant1/1 -> Product2/2
  Abs1/1 -> Add2/2
  Abs/1 -> Add2/1
  In3/1 -> Product5/2
  Product5/1 -> Add1/1
  Constant2/1 -> Product3/2
  Product3/1 -> Sum2/1
  Clock 2/1(q) -> Sum2/2
  fpga_dfe/1(q) -> Product/1
  fpga_dfe1/1(q) -> Product1/1
  Add1/1 -> Delay6/1
  Constant3/1 -> Switch/3
  Counter/1 -> Switch/2
  Pulse Generator2/1 -> Counter/1
  Sum2/1 -> Clock 1/2(d)
  Clock 1/1(q) -> Product5/1, Sum1/2, Clock 2/2(d)
  Delay/1 -> Switch/1
  fpga_dfe2/1(q) -> q/1
  fpga_dfe3/1(q) -> Out2/1
  Add2/1 -> Clock 5/2(d)
  Clock 5/1(q) -> Sum1/1
  In1/1 -> fpga_dfe/2(d)
  In2/1 -> fpga_dfe1/2(d)
  Delay8/1 -> fpga_dfe3/2(d), Abs/1
  Delay9/1 -> Abs1/1, fpga_dfe2/2(d)
  Sum1/1 -> Delay3/1
  Delay3/1 -> Product3/1
  Delay4/1 -> Delay12/1, Delay13/1, Clock 1/1(ena)
  Delay13/1 -> Clock 2/1(ena)
  Delay6/1 -> Product2/1
  Delay5/1 -> Delay7/1, Clock 4/1(ena)
  Delay7/1 -> fpga_dfe3/1(ena), fpga_dfe2/1(ena)
  ena/1 -> Delay10/1, fpga_dfe1/1(ena), fpga_dfe/1(ena)
  Delay10/1 -> Delay11/1
  Delay11/1 -> Delay1/1, Clock 5/1(ena)
  Delay1/1 -> Delay4/1
  Delay12/1 -> Delay5/1

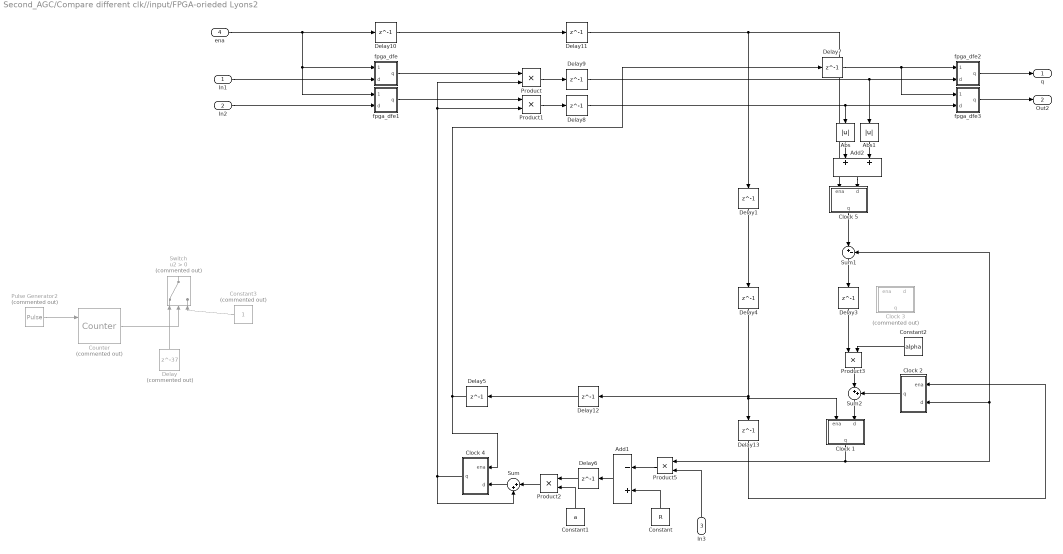
== system Second_AGC/Compare different clk//input/FPGA-orieded Lyons2 ==
  In1 : Inport
  In2 : Inport  Port=2
  In3 : Inport  Port=3
  ena : Inport  Port=4
  Abs : Abs  SaturateOnIntegerOverflow=off
  Abs1 : Abs  SaturateOnIntegerOverflow=off
  Add1 : Sum  Inputs=-+  AccumDataTypeStr=double
  Add2 : Sum  AccumDataTypeStr=double
  Clock 1 : Subsystem
  Clock 2 : Subsystem
  Clock 3 : Subsystem  Commented=on
  Clock 4 : Subsystem
  Clock 5 : Subsystem
  Constant : Constant  Value=R  SampleTime=-1
  Constant1 : Constant  Value=a  SampleTime=-1
  Constant2 : Constant  Value=alpha  SampleTime=-1
  Constant3 : Constant  Commented=on  SampleTime=-1
  Counter : dspswit3/Counter  Commented=on  Direction=Up  CountEvent=Rising edge  CounterSize=User defined  MaxCount=1  InitialCount=0  Output=Count  HitValue=32  ResetInput=on  SamplesPerFrame=1  Ts=1  CntDtype=double  HitDtype=Logical
  Delay : Delay  Commented=on  DelayLength=37  InitialCondition=0
  Delay{1,3..13} (12 alike) : Delay  DelayLength=1  InitialCondition=0
  Product{,1..3,5} (5 alike) : Product  OutDataTypeStr=double
  Pulse Generator2 : DiscretePulseGenerator  Commented=on  PulseType=Time based  Period=Time*20000  PulseWidth=50  PhaseDelay=41
  Sum : Sum  Inputs=|++  AccumDataTypeStr=double
  Sum1 : Sum  Inputs=|+-  AccumDataTypeStr=double
  Sum2 : Sum  Inputs=|++  AccumDataTypeStr=double
  Switch : Switch  Commented=on  Criteria=u2 > Threshold  SaturateOnIntegerOverflow=off  InputSameDT=off
  fpga_dfe : Subsystem  AncestorBlock=sim_stud_lib_r2022a/fpga_dfe
      mask Display:
      | disp('D');
      | port_label('input',1,'e');
      | port_label('input',2,'d');
      | port_label('output',1,'q');
  fpga_dfe1 : Subsystem  AncestorBlock=sim_stud_lib_r2022a/fpga_dfe
      mask Display:
      | disp('D');
      | port_label('input',1,'e');
      | port_label('input',2,'d');
      | port_label('output',1,'q');
  fpga_dfe2 : Subsystem  AncestorBlock=sim_stud_lib_r2022a/fpga_dfe
      mask Display:
      | disp('D');
      | port_label('input',1,'e');
      | port_label('input',2,'d');
      | port_label('output',1,'q');
  fpga_dfe3 : Subsystem  AncestorBlock=sim_stud_lib_r2022a/fpga_dfe
      mask Display:
      | disp('D');
      | port_label('input',1,'e');
      | port_label('input',2,'d');
      | port_label('output',1,'q');
  q : Outport
  Out2 : Outport  Port=2
  wires:
  Clock 4/1(q) -> Sum/2, Product1/2, Product/2
  Product/1 -> Delay9/1
  Product1/1 -> Delay8/1
  Constant/1 -> Add1/2
  Sum/1 -> Clock 4/2(d)
  Product2/1 -> Sum/1
  Constant1/1 -> Product2/2
  Abs1/1 -> Add2/2
  Abs/1 -> Add2/1
  In3/1 -> Product5/2
  Product5/1 -> Add1/1
  Constant2/1 -> Product3/2
  Product3/1 -> Sum2/1
  Clock 2/1(q) -> Sum2/2
  fpga_dfe/1(q) -> Product/1
  fpga_dfe1/1(q) -> Product1/1
  Add1/1 -> Delay6/1
  Constant3/1 -> Switch/3
  Counter/1 -> Switch/2
  Pulse Generator2/1 -> Counter/1
  Sum2/1 -> Clock 1/2(d)
  Clock 1/1(q) -> Product5/1, Sum1/2, Clock 2/2(d)
  Delay/1 -> Switch/1
  fpga_dfe2/1(q) -> q/1
  fpga_dfe3/1(q) -> Out2/1
  Add2/1 -> Clock 5/2(d)
  Clock 5/1(q) -> Sum1/1
  In1/1 -> fpga_dfe/2(d)
  In2/1 -> fpga_dfe1/2(d)
  Delay8/1 -> fpga_dfe3/2(d), Abs/1
  Delay9/1 -> Abs1/1, fpga_dfe2/2(d)
  Sum1/1 -> Delay3/1
  Delay3/1 -> Product3/1
  Delay4/1 -> Delay12/1, Delay13/1, Clock 1/1(ena)
  Delay13/1 -> Clock 2/1(ena)
  Delay6/1 -> Product2/1
  Delay5/1 -> Delay7/1, Clock 4/1(ena)
  Delay7/1 -> fpga_dfe3/1(ena), fpga_dfe2/1(ena)
  ena/1 -> Delay10/1, fpga_dfe1/1(ena), fpga_dfe/1(ena)
  Delay10/1 -> Delay11/1
  Delay11/1 -> Delay1/1, Clock 5/1(ena)
  Delay1/1 -> Delay4/1
  Delay12/1 -> Delay5/1

== system Second_AGC/FPGA-orieded Lyons/Clock 1 ==
  ena : Inport
  d : Inport  Port=2
  Delay16 : Delay  DelayLength=1
  Enabled Subsystem : sim_stud_lib_r2022a/fpga_dfe/Enabled Subsystem  SystemSampleTime=-1  VariantActivationTime=update diagram  Latency=0  AutoFrameSizeCalculation=off
  q : Outport  VectorParamsAs1DForOutWhenUnconnected=off
  wires:
  Delay16/1 -> q/1
  d/1 -> Enabled Subsystem/1
  Enabled Subsystem/1 -> Delay16/1
  ena/1 -> Enabled Subsystem/Enable

== system Second_AGC/FPGA-orieded Lyons/Clock 2 ==
  ena : Inport
  d : Inport  Port=2
  Delay16 : Delay  DelayLength=1
  Enabled Subsystem : sim_stud_lib_r2022a/fpga_dfe/Enabled Subsystem  SystemSampleTime=-1  VariantActivationTime=update diagram  Latency=0  AutoFrameSizeCalculation=off
  q : Outport  VectorParamsAs1DForOutWhenUnconnected=off
  wires:
  Delay16/1 -> q/1
  d/1 -> Enabled Subsystem/1
  Enabled Subsystem/1 -> Delay16/1
  ena/1 -> Enabled Subsystem/Enable

== system Second_AGC/FPGA-orieded Lyons/Clock 3 ==
  ena : Inport
  d : Inport  Port=2
  Delay16 : Delay  DelayLength=1
  Enabled Subsystem : sim_stud_lib_r2022a/fpga_dfe/Enabled Subsystem  SystemSampleTime=-1  VariantActivationTime=update diagram  Latency=0  AutoFrameSizeCalculation=off
  q : Outport  VectorParamsAs1DForOutWhenUnconnected=off
  wires:
  Delay16/1 -> q/1
  d/1 -> Enabled Subsystem/1
  Enabled Subsystem/1 -> Delay16/1
  ena/1 -> Enabled Subsystem/Enable

== system Second_AGC/FPGA-orieded Lyons/Clock 4 ==
  ena : Inport
  d : Inport  Port=2
  Delay16 : Delay  DelayLength=1
  Enabled Subsystem : sim_stud_lib_r2022a/fpga_dfe/Enabled Subsystem  SystemSampleTime=-1  VariantActivationTime=update diagram  Latency=0  AutoFrameSizeCalculation=off
  q : Outport  VectorParamsAs1DForOutWhenUnconnected=off
  wires:
  Delay16/1 -> q/1
  d/1 -> Enabled Subsystem/1
  Enabled Subsystem/1 -> Delay16/1
  ena/1 -> Enabled Subsystem/Enable

== system Second_AGC/FPGA-orieded Lyons/Clock 5 ==
  ena : Inport
  d : Inport  Port=2
  Delay16 : Delay  DelayLength=1
  Enabled Subsystem : sim_stud_lib_r2022a/fpga_dfe/Enabled Subsystem  SystemSampleTime=-1  VariantActivationTime=update diagram  Latency=0  AutoFrameSizeCalculation=off
  q : Outport  VectorParamsAs1DForOutWhenUnconnected=off
  wires:
  Delay16/1 -> q/1
  d/1 -> Enabled Subsystem/1
  Enabled Subsystem/1 -> Delay16/1
  ena/1 -> Enabled Subsystem/Enable

== system Second_AGC/FPGA-orieded Lyons/fpga_dfe ==
  ena : Inport
  d : Inport  Port=2
  Delay16 : Delay  DelayLength=1
  Enabled Subsystem : Subsystem  TreatAsAtomicUnit=on
  q : Outport  VectorParamsAs1DForOutWhenUnconnected=off
  wires:
  Enabled Subsystem/1(Out1) -> Delay16/1
  Delay16/1 -> q/1
  ena/1 -> Enabled Subsystem/Enable
  d/1 -> Enabled Subsystem/1(In1)

== system Second_AGC/FPGA-orieded Lyons/fpga_dfe1 ==
  ena : Inport
  d : Inport  Port=2
  Delay16 : Delay  DelayLength=1
  Enabled Subsystem : Subsystem  TreatAsAtomicUnit=on
  q : Outport  VectorParamsAs1DForOutWhenUnconnected=off
  wires:
  Enabled Subsystem/1(Out1) -> Delay16/1
  Delay16/1 -> q/1
  ena/1 -> Enabled Subsystem/Enable
  d/1 -> Enabled Subsystem/1(In1)

== system Second_AGC/FPGA-orieded Lyons/fpga_dfe2 ==
  ena : Inport
  d : Inport  Port=2
  Delay16 : Delay  DelayLength=1
  Enabled Subsystem : Subsystem  TreatAsAtomicUnit=on
  q : Outport  VectorParamsAs1DForOutWhenUnconnected=off
  wires:
  Enabled Subsystem/1(Out1) -> Delay16/1
  Delay16/1 -> q/1
  ena/1 -> Enabled Subsystem/Enable
  d/1 -> Enabled Subsystem/1(In1)

== system Second_AGC/FPGA-orieded Lyons/fpga_dfe3 ==
  ena : Inport
  d : Inport  Port=2
  Delay16 : Delay  DelayLength=1
  Enabled Subsystem : Subsystem  TreatAsAtomicUnit=on
  q : Outport  VectorParamsAs1DForOutWhenUnconnected=off
  wires:
  Enabled Subsystem/1(Out1) -> Delay16/1
  Delay16/1 -> q/1
  ena/1 -> Enabled Subsystem/Enable
  d/1 -> Enabled Subsystem/1(In1)

== system Second_AGC/Fixed Point FPGA-oriended Lyons/Clock 1 ==
  ena : Inport
  d : Inport  Port=2
  Delay16 : Delay  DelayLength=1
  Enabled Subsystem : sim_stud_lib_r2022a/fpga_dfe/Enabled Subsystem  SystemSampleTime=-1  VariantActivationTime=update diagram  Latency=0  AutoFrameSizeCalculation=off
  q : Outport  VectorParamsAs1DForOutWhenUnconnected=off
  wires:
  Delay16/1 -> q/1
  d/1 -> Enabled Subsystem/1
  Enabled Subsystem/1 -> Delay16/1
  ena/1 -> Enabled Subsystem/Enable

== system Second_AGC/Fixed Point FPGA-oriended Lyons/Clock 2 ==
  ena : Inport
  d : Inport  Port=2
  Delay16 : Delay  DelayLength=1
  Enabled Subsystem : sim_stud_lib_r2022a/fpga_dfe/Enabled Subsystem  SystemSampleTime=-1  VariantActivationTime=update diagram  Latency=0  AutoFrameSizeCalculation=off
  q : Outport  VectorParamsAs1DForOutWhenUnconnected=off
  wires:
  Delay16/1 -> q/1
  d/1 -> Enabled Subsystem/1
  Enabled Subsystem/1 -> Delay16/1
  ena/1 -> Enabled Subsystem/Enable

== system Second_AGC/Fixed Point FPGA-oriended Lyons/Clock 3 ==
  ena : Inport
  d : Inport  Port=2
  Delay16 : Delay  DelayLength=1
  Enabled Subsystem : sim_stud_lib_r2022a/fpga_dfe/Enabled Subsystem  SystemSampleTime=-1  VariantActivationTime=update diagram  Latency=0  AutoFrameSizeCalculation=off
  q : Outport  VectorParamsAs1DForOutWhenUnconnected=off
  wires:
  Delay16/1 -> q/1
  d/1 -> Enabled Subsystem/1
  Enabled Subsystem/1 -> Delay16/1
  ena/1 -> Enabled Subsystem/Enable

== system Second_AGC/Fixed Point FPGA-oriended Lyons/Clock 4 ==
  ena : Inport
  d : Inport  Port=2
  Delay16 : Delay  DelayLength=1
  Enabled Subsystem : sim_stud_lib_r2022a/fpga_dfe/Enabled Subsystem  SystemSampleTime=-1  VariantActivationTime=update diagram  Latency=0  AutoFrameSizeCalculation=off
  q : Outport  VectorParamsAs1DForOutWhenUnconnected=off
  wires:
  Delay16/1 -> q/1
  d/1 -> Enabled Subsystem/1
  Enabled Subsystem/1 -> Delay16/1
  ena/1 -> Enabled Subsystem/Enable

== system Second_AGC/Fixed Point FPGA-oriended Lyons/Clock 5 ==
  ena : Inport
  d : Inport  Port=2
  Delay16 : Delay  DelayLength=1
  Enabled Subsystem : sim_stud_lib_r2022a/fpga_dfe/Enabled Subsystem  SystemSampleTime=-1  VariantActivationTime=update diagram  Latency=0  AutoFrameSizeCalculation=off
  q : Outport  VectorParamsAs1DForOutWhenUnconnected=off
  wires:
  Delay16/1 -> q/1
  d/1 -> Enabled Subsystem/1
  Enabled Subsystem/1 -> Delay16/1
  ena/1 -> Enabled Subsystem/Enable

== system Second_AGC/Fixed Point FPGA-oriended Lyons/fpga_dfe ==
  ena : Inport
  d : Inport  Port=2
  Delay16 : Delay  DelayLength=1
  Enabled Subsystem : Subsystem  TreatAsAtomicUnit=on
  q : Outport  VectorParamsAs1DForOutWhenUnconnected=off
  wires:
  Enabled Subsystem/1(Out1) -> Delay16/1
  Delay16/1 -> q/1
  ena/1 -> Enabled Subsystem/Enable
  d/1 -> Enabled Subsystem/1(In1)

== system Second_AGC/Fixed Point FPGA-oriended Lyons/fpga_dfe1 ==
  ena : Inport
  d : Inport  Port=2
  Delay16 : Delay  DelayLength=1
  Enabled Subsystem : Subsystem  TreatAsAtomicUnit=on
  q : Outport  VectorParamsAs1DForOutWhenUnconnected=off
  wires:
  Enabled Subsystem/1(Out1) -> Delay16/1
  Delay16/1 -> q/1
  ena/1 -> Enabled Subsystem/Enable
  d/1 -> Enabled Subsystem/1(In1)

== system Second_AGC/Fixed Point FPGA-oriended Lyons/fpga_dfe2 ==
  ena : Inport
  d : Inport  Port=2
  Delay16 : Delay  DelayLength=1
  Enabled Subsystem : Subsystem  TreatAsAtomicUnit=on
  q : Outport  VectorParamsAs1DForOutWhenUnconnected=off
  wires:
  Enabled Subsystem/1(Out1) -> Delay16/1
  Delay16/1 -> q/1
  ena/1 -> Enabled Subsystem/Enable
  d/1 -> Enabled Subsystem/1(In1)

== system Second_AGC/Fixed Point FPGA-oriended Lyons/fpga_dfe3 ==
  ena : Inport
  d : Inport  Port=2
  Delay16 : Delay  DelayLength=1
  Enabled Subsystem : Subsystem  TreatAsAtomicUnit=on
  q : Outport  VectorParamsAs1DForOutWhenUnconnected=off
  wires:
  Enabled Subsystem/1(Out1) -> Delay16/1
  Delay16/1 -> q/1
  ena/1 -> Enabled Subsystem/Enable
  d/1 -> Enabled Subsystem/1(In1)

== system Second_AGC/Calculation of average power/MA and divide AGC/fpga_dfe2 ==
  ena : Inport
  d : Inport  Port=2
  Delay16 : Delay  DelayLength=1
  Enabled Subsystem : Subsystem  TreatAsAtomicUnit=on
  q : Outport  VectorParamsAs1DForOutWhenUnconnected=off
  wires:
  Enabled Subsystem/1(Out1) -> Delay16/1
  Delay16/1 -> q/1
  ena/1 -> Enabled Subsystem/Enable
  d/1 -> Enabled Subsystem/1(In1)

== system Second_AGC/Calculation of average power/MA and divide AGC/fpga_dfe3 ==
  ena : Inport
  d : Inport  Port=2
  Delay16 : Delay  DelayLength=1
  Enabled Subsystem : Subsystem  TreatAsAtomicUnit=on
  q : Outport  VectorParamsAs1DForOutWhenUnconnected=off
  wires:
  Enabled Subsystem/1(Out1) -> Delay16/1
  Delay16/1 -> q/1
  ena/1 -> Enabled Subsystem/Enable
  d/1 -> Enabled Subsystem/1(In1)

== system Second_AGC/Calculation of average power/MA and divide input /fpga_dfe2 ==
  ena : Inport
  d : Inport  Port=2
  Delay16 : Delay  DelayLength=1
  Enabled Subsystem : Subsystem  TreatAsAtomicUnit=on
  q : Outport  VectorParamsAs1DForOutWhenUnconnected=off
  wires:
  Enabled Subsystem/1(Out1) -> Delay16/1
  Delay16/1 -> q/1
  ena/1 -> Enabled Subsystem/Enable
  d/1 -> Enabled Subsystem/1(In1)

== system Second_AGC/Calculation of average power/MA and divide input /fpga_dfe3 ==
  ena : Inport
  d : Inport  Port=2
  Delay16 : Delay  DelayLength=1
  Enabled Subsystem : Subsystem  TreatAsAtomicUnit=on
  q : Outport  VectorParamsAs1DForOutWhenUnconnected=off
  wires:
  Enabled Subsystem/1(Out1) -> Delay16/1
  Delay16/1 -> q/1
  ena/1 -> Enabled Subsystem/Enable
  d/1 -> Enabled Subsystem/1(In1)

== system Second_AGC/Calculation of average power1/MA and divide AGC/fpga_dfe2 ==
  ena : Inport
  d : Inport  Port=2
  Delay16 : Delay  DelayLength=1
  Enabled Subsystem : Subsystem  TreatAsAtomicUnit=on
  q : Outport  VectorParamsAs1DForOutWhenUnconnected=off
  wires:
  Enabled Subsystem/1(Out1) -> Delay16/1
  Delay16/1 -> q/1
  ena/1 -> Enabled Subsystem/Enable
  d/1 -> Enabled Subsystem/1(In1)

== system Second_AGC/Calculation of average power1/MA and divide AGC/fpga_dfe3 ==
  ena : Inport
  d : Inport  Port=2
  Delay16 : Delay  DelayLength=1
  Enabled Subsystem : Subsystem  TreatAsAtomicUnit=on
  q : Outport  VectorParamsAs1DForOutWhenUnconnected=off
  wires:
  Enabled Subsystem/1(Out1) -> Delay16/1
  Delay16/1 -> q/1
  ena/1 -> Enabled Subsystem/Enable
  d/1 -> Enabled Subsystem/1(In1)

== system Second_AGC/Calculation of average power1/MA and divide input /fpga_dfe2 ==
  ena : Inport
  d : Inport  Port=2
  Delay16 : Delay  DelayLength=1
  Enabled Subsystem : Subsystem  TreatAsAtomicUnit=on
  q : Outport  VectorParamsAs1DForOutWhenUnconnected=off
  wires:
  Enabled Subsystem/1(Out1) -> Delay16/1
  Delay16/1 -> q/1
  ena/1 -> Enabled Subsystem/Enable
  d/1 -> Enabled Subsystem/1(In1)
